simulink model "openLoop"  (R2021b)
settings: Solver=VariableStepAuto  StartTime=0.0  StopTime=857  RelTol=1e-3
settings Model: Creator=Asus  LastModifiedBy=Asus

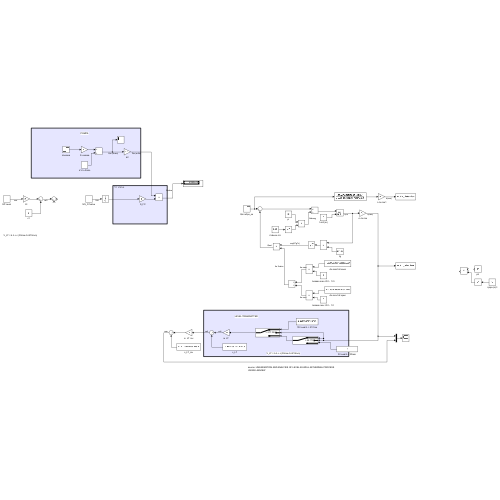
[thumbnail: Simulink's stored preview of the top-level diagram]
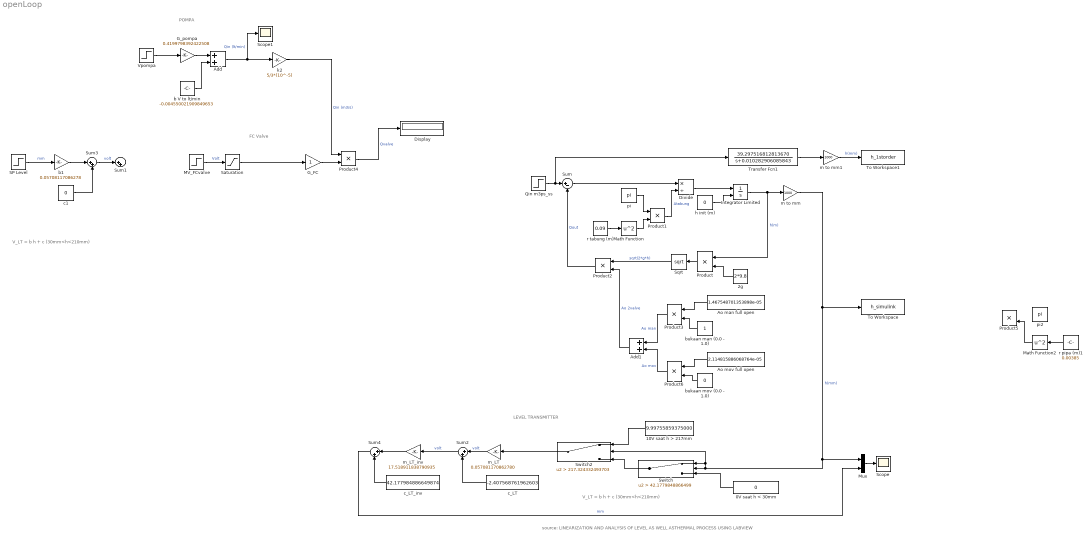
== system openLoop ==
  note: V_LT = b h + c (30mm<h<210mm)
  note: LEVEL TRANSMITTER
  note: FC Valve
  note: POMPA
  note: source: LINEARIZATION AND ANALYSIS OF LEVEL AS WELL ASTHERMAL PROCESS USING LABVIEW
  note: V_LT = b h + c (30mm<h<210mm)
  0V saat h < 30mm : Constant  Value=0
  10V saat h > 217mm : Constant  Value=9.99755859375000
  2g : Constant  Value=2*9.8
  Add : Sum
  Add1 : Sum
  Ao man full open : Constant  Value=1.467548701353898e-05
  Ao mov full open : Constant  Value=2.114815886068764e-05
  Display : Display
  Divide : Product  Inputs=*/
  G_FC : Gain
  G_pompa : Gain  Gain=0.4199798392422508
  Integrator Limited : Integrator  InitialConditionSource=external  LimitOutput=on  UpperSaturationLimit=1  LowerSaturationLimit=0
  MV_FCvalve : Step  SampleTime=0
  Math Function : Math  Operator=square  SaturateOnIntegerOverflow=on
  Math Function2 : Math  Operator=square  SaturateOnIntegerOverflow=on
  Mux : Mux  Inputs=2
  Product{,1..6} (7 alike) : Product
  Qin m3ps_ss : Step  After=1.613207956317757e-05  SampleTime=0.05
  SP Level : Step  SampleTime=0
  Saturation : Saturate  UpperLimit=10  LowerLimit=0
  Scope : Scope
  Scope1 : Scope
  Sqrt : Sqrt  SaturateOnIntegerOverflow=on
  Sum : Sum  Inputs=|+-
  Sum{1..4} (4 alike) : Sum  Inputs=|++
  Switch : Switch  Criteria=u2 > Threshold  Threshold=42.1779848866499
  Switch2 : Switch  Criteria=u2 > Threshold  Threshold=217.324332493703
  To Workspace : ToWorkspace  VariableName=h_simulink  SampleTime=-1
  To Workspace1 : ToWorkspace  VariableName=h_1storder  SampleTime=-1
      settings: Save2DSignal=2-D array (concatenate along first dimension)
  Transfer Fcn1 : TransferFcn  Numerator=[39.297516812813670]  Denominator=[1 0.010282906085843]
  Vpompa : Step  After=10  SampleTime=0
  b V to lt/min : Constant  Value=-0.004550021909849653
  b1 : Gain  Gain=0.05708117086278
  bukaan man (0.0 - 1.0) : Constant
  bukaan mov (0.0 - 1.0) : Constant  Value=0
  c1 : Constant  Value=0
  c_LT : Constant  Value=-2.407568761962603
  c_LT_inv : Constant  Value=42.177984886649874
  h init (m) : Constant  Value=0
  k2 : Gain  Gain=5/3*(10^-5)
  m to mm : Gain  Gain=1000
  m to mm1 : Gain  Gain=1000
  m_LT : Gain  Gain=0.057081170862780
  m_LT_inv : Gain  Gain=17.518911838790935
  pi : Constant  Value=pi
  pi2 : Constant  Value=pi
  r pipa (m)1 : Constant  Value=0.00385
  r tabung (m) : Constant  Value=0.09
  wires:
  Divide/1 -> Integrator Limited/1
  Product/1 -> Sqrt/1
  2g/1 -> Product/2
  Sqrt/1 -> Product2/1  "sqrt(2*g*h)"
  h init (m)/1 -> Integrator Limited/2
  Product1/1 -> Divide/2  "Atabung"
  pi/1 -> Product1/1
  Math Function/1 -> Product1/2
  r tabung (m)/1 -> Math Function/1
  Add1/1 -> Product2/2  "Ao 2valve"
  G_pompa/1 -> Add/1
  Add/1 -> Scope1/1, k2/1  "Qin (lt/min)"
  b V to lt/min/1 -> Add/2
  k2/1 -> Product4/1  "Qin (m3/s)"
  Product4/1 -> Display/1  "Qvalve"
  MV_FCvalve/1 -> Saturation/1  "Volt"
  G_FC/1 -> Product4/2
  SP Level/1 -> b1/1  "mm"
  b1/1 -> Sum3/1
  Integrator Limited/1 -> Product/1, m to mm/1  "h(m)"
  m to mm/1 -> To Workspace/1, Mux/1, Switch2/2, Switch/1, Switch/2  "h(mm)"
  Vpompa/1 -> G_pompa/1
  Saturation/1 -> G_FC/1
  0V saat h < 30mm/1 -> Switch/3
  Switch/1 -> Switch2/3
  10V saat h > 217mm/1 -> Switch2/1
  Switch2/1 -> m_LT/1
  m_LT/1 -> Sum2/1  "volt"
  c_LT/1 -> Sum2/2
  c1/1 -> Sum3/2
  Sum3/1 -> Sum1/1  "volt"
  Sum2/1 -> m_LT_inv/1  "volt"
  m_LT_inv/1 -> Sum4/1
  c_LT_inv/1 -> Sum4/2
  Sum4/1 -> Mux/2  "mm"
  Mux/1 -> Scope/1
  Math Function2/1 -> Product5/2
  r pipa (m)1/1 -> Math Function2/1
  Ao man full open/1 -> Product3/1
  Product3/1 -> Add1/1  "Ao man"
  Product6/1 -> Add1/2  "Ao mov"
  Ao mov full open/1 -> Product6/1
  bukaan man (0.0 - 1.0)/1 -> Product3/2
  bukaan mov (0.0 - 1.0)/1 -> Product6/2
  Sum/1 -> Divide/1
  Product2/1 -> Sum/2  "Qout"
  Qin m3ps_ss/1 -> Transfer Fcn1/1, Sum/1
  Transfer Fcn1/1 -> m to mm1/1
  m to mm1/1 -> To Workspace1/1  "h(mm)"
